simulink subsystem "saturation_range"  (R2020b)
settings: Solver=VariableStepAuto  StartTime=0.0  StopTime=10.0  RelTol=1e-3
settings Model: Creator=RH  LastModifiedBy=Marco

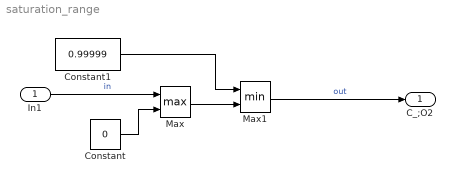
== system saturation_range ==
  In1 : Inport
  Constant : Constant  Value=0
  Constant1 : Constant  Value=0.99999
  Max : MinMax  Function=max  Inputs=2
  Max1 : MinMax  Inputs=2
  C_;O2 : Outport
  wires:
  Max1/1 -> C_;O2/1  "out"
  Constant/1 -> Max/2
  Max/1 -> Max1/2
  Constant1/1 -> Max1/1
  In1/1 -> Max/1  "in"
